simulink model "ball_pipe_nonlinear"  (R2025b)
settings: Solver=ode4  StartTime=0.0  StopTime=14  FixedStep=0.0003333333333333333  RelTol=1e-3
values from neighbouring files (symbols this model uses):
  bp = ball_pipe_defaults()    [analyze_two_link_mechanism.m]    (also in build_ball_pipe_model.m; run_ball_pipe_demo.m; run_ball_pipe_sweep.m = scenarios(index); run_camera_rate_comparison.m = scenarios(scenario_index))
settings Model: Creator=ASUS  LastModifiedBy=ASUS

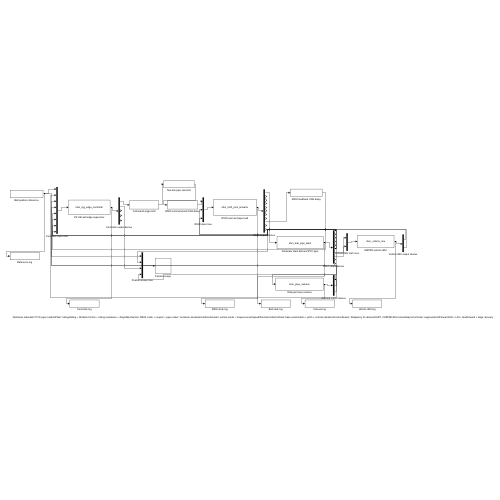
[thumbnail: Simulink's stored preview of the top-level diagram]
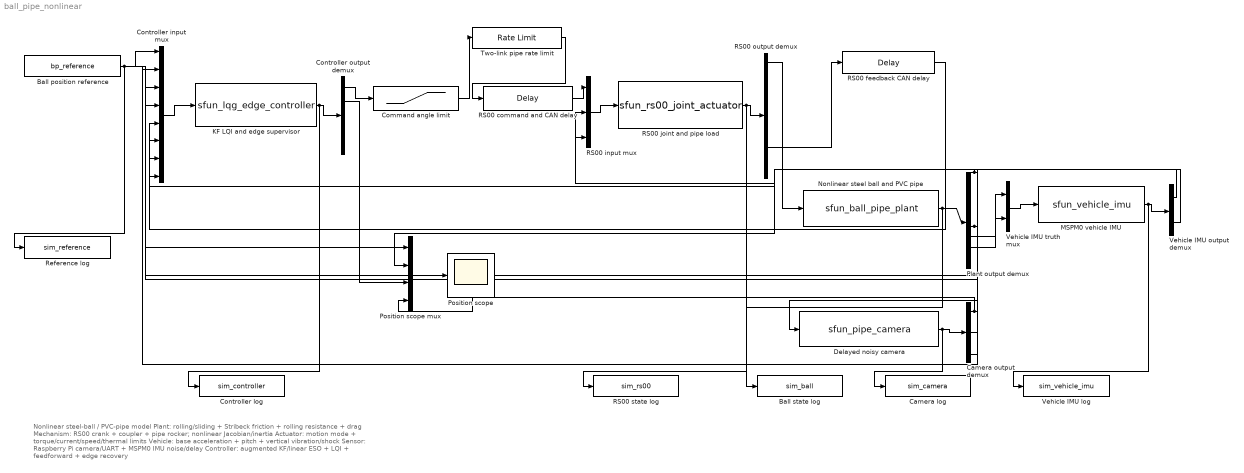
== system ball_pipe_nonlinear ==
  note: Nonlinear steel-ball / PVC-pipe model\nPlant: rolling/sliding + Stribeck friction + rolling resistance + drag\nMechanism: RS00 crank + coupler + pipe rocker; nonlinear Jacobian/inertia\nActuator: motion mode + torque/current/speed/thermal limits\nVehicle: base acceleration + pitch + vertical vibration/shock\nSensor: Raspberry Pi camera/UART + MSPM0 IMU noise/delay\nController: augmented KF/linear ESO + LQI + feedforward + edge recovery
  Ball position reference : FromWorkspace  VariableName=bp_reference  Interpolate=off  OutputAfterFinalValue=Holding final value
  Ball state log : ToWorkspace  VariableName=sim_ball  SaveFormat=Timeseries  SampleTime=-1
  Camera log : ToWorkspace  VariableName=sim_camera  SaveFormat=Timeseries  SampleTime=-1
  Camera output demux : Demux  Outputs=3
  Command angle limit : Saturate  UpperLimit=bp.actuator.max_angle  LowerLimit=-bp.actuator.max_angle
  Controller input mux : Mux  Inputs=8
  Controller log : ToWorkspace  VariableName=sim_controller  SaveFormat=Timeseries  SampleTime=-1
  Controller output demux : Demux  Outputs=5
  Delayed noisy camera : M-S-Function  FunctionName=sfun_pipe_camera  Parameters=bp
  KF LQI and edge supervisor : M-S-Function  FunctionName=sfun_lqg_edge_controller  Parameters=bp
  MSPM0 vehicle IMU : M-S-Function  FunctionName=sfun_vehicle_imu  Parameters=bp
  Nonlinear steel ball and PVC pipe : M-S-Function  FunctionName=sfun_ball_pipe_plant  Parameters=bp
  Plant output demux : Demux  Outputs=10
  Position scope : Scope
  Position scope mux : Mux
  RS00 command and CAN delay : TransportDelay  DelayTime=bp.actuator.delay
  RS00 feedback CAN delay : TransportDelay  DelayTime=bp.rs00.feedback_delay
  RS00 input mux : Mux  Inputs=3
  RS00 joint and pipe load : M-S-Function  FunctionName=sfun_rs00_joint_actuator  Parameters=bp
  RS00 output demux : Demux  Outputs=11
  RS00 state log : ToWorkspace  VariableName=sim_rs00  SaveFormat=Timeseries  SampleTime=-1
  Reference log : ToWorkspace  VariableName=sim_reference  SaveFormat=Timeseries  SampleTime=-1
  Two-link pipe rate limit : RateLimiter  RisingSlewLimit=bp.actuator.max_rate  FallingSlewLimit=-bp.actuator.max_rate  SampleTimeMode=inherited
  Vehicle IMU log : ToWorkspace  VariableName=sim_vehicle_imu  SaveFormat=Timeseries  SampleTime=-1
  Vehicle IMU output demux : Demux  Outputs=2
  Vehicle IMU truth mux : Mux  Inputs=2
  wires:
  Ball position reference/1 -> Controller input mux/1, Position scope mux/1, Reference log/1
  Controller input mux/1 -> KF LQI and edge supervisor/1
  KF LQI and edge supervisor/1 -> Controller output demux/1, Controller log/1
  Controller output demux/1 -> Command angle limit/1
  Command angle limit/1 -> Two-link pipe rate limit/1
  Two-link pipe rate limit/1 -> RS00 command and CAN delay/1
  RS00 command and CAN delay/1 -> RS00 input mux/1
  RS00 input mux/1 -> RS00 joint and pipe load/1
  RS00 joint and pipe load/1 -> RS00 output demux/1, RS00 state log/1
  RS00 output demux/1 -> Nonlinear steel ball and PVC pipe/1
  RS00 output demux/9 -> RS00 feedback CAN delay/1
  RS00 feedback CAN delay/1 -> Controller input mux/5
  Nonlinear steel ball and PVC pipe/1 -> Plant output demux/1, Ball state log/1
  Plant output demux/1 -> RS00 input mux/2, Delayed noisy camera/1, Position scope mux/2
  Plant output demux/6 -> Controller input mux/6, RS00 input mux/3
  Plant output demux/7 -> Vehicle IMU truth mux/1
  Plant output demux/8 -> Vehicle IMU truth mux/2
  Vehicle IMU truth mux/1 -> MSPM0 vehicle IMU/1
  MSPM0 vehicle IMU/1 -> Vehicle IMU output demux/1, Vehicle IMU log/1
  Vehicle IMU output demux/1 -> Controller input mux/7
  Vehicle IMU output demux/2 -> Controller input mux/8
  Delayed noisy camera/1 -> Camera output demux/1, Camera log/1
  Camera output demux/1 -> Controller input mux/2, Position scope mux/4
  Camera output demux/2 -> Controller input mux/3
  Camera output demux/3 -> Controller input mux/4
  Controller output demux/2 -> Position scope mux/3
  Position scope mux/1 -> Position scope/1
